simulink subsystem "Automatic_turn_light_feature_continuous_mdl"  (R2026a)
settings: Solver=VariableStepAuto
settings Model: Creator=irfan  LastModifiedBy=irfan

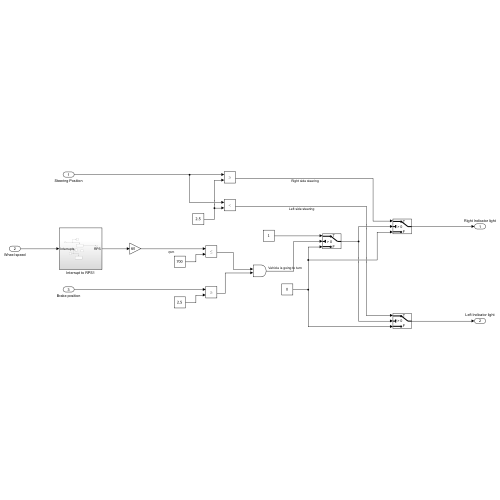
[thumbnail: Simulink's stored preview of the top-level diagram]
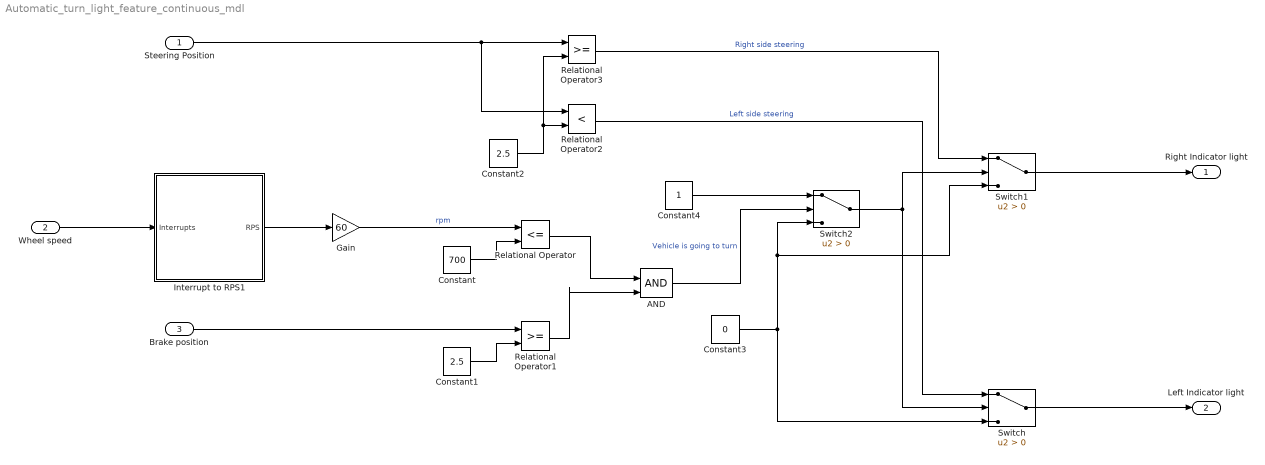
== system Automatic_turn_light_feature_continuous_mdl ==
  Steering Position : Inport
  Wheel speed : Inport  Port=2
  Brake position : Inport  Port=3
  AND : Logic  IconShape=distinctive  AllPortsSameDT=off  OutDataTypeStr=boolean
  Constant : Constant  Value=700
  Constant1 : Constant  Value=2.5
  Constant2 : Constant  Value=2.5
  Constant3 : Constant  Value=0
  Constant4 : Constant
  Gain : Gain  Gain=60
  Interrupt to RPS1 : Subsystem
  Relational Operator : RelationalOperator  Operator=<=  OutDataTypeStr=boolean  RndMeth=Simplest  InputSameDT=off
  Relational Operator1 : RelationalOperator  OutDataTypeStr=boolean  RndMeth=Simplest  InputSameDT=off
  Relational Operator2 : RelationalOperator  Operator=<  OutDataTypeStr=boolean  RndMeth=Simplest  InputSameDT=off
  Relational Operator3 : RelationalOperator  OutDataTypeStr=boolean  RndMeth=Simplest  InputSameDT=off
  Switch : Switch  Criteria=u2 > Threshold  SaturateOnIntegerOverflow=off  InputSameDT=off
  Switch1 : Switch  Criteria=u2 > Threshold  SaturateOnIntegerOverflow=off  InputSameDT=off
  Switch2 : Switch  Criteria=u2 > Threshold  SaturateOnIntegerOverflow=off  InputSameDT=off
  Right Indicator light : Outport
  Left Indicator light : Outport  Port=2
  wires:
  Relational Operator2/1 -> Switch/1  "Left side steering"
  Relational Operator1/1 -> AND/2
  Steering Position/1 -> Relational Operator3/1, Relational Operator2/1
  Constant2/1 -> Relational Operator2/2, Relational Operator3/2
  AND/1 -> Switch2/2  "Vehicle is going to turn"
  Constant3/1 -> Switch/3, Switch1/3, Switch2/3
  Constant4/1 -> Switch2/1
  Constant1/1 -> Relational Operator1/2
  Switch2/1 -> Switch/2, Switch1/2
  Constant/1 -> Relational Operator/2
  Gain/1 -> Relational Operator/1  "rpm"
  Relational Operator3/1 -> Switch1/1  "Right side steering"
  Relational Operator/1 -> AND/1
  Switch/1 -> Left Indicator light/1
  Switch1/1 -> Right Indicator light/1
  Brake position/1 -> Relational Operator1/1
  Wheel speed/1 -> Interrupt to RPS1/1(Interrupts)
  Interrupt to RPS1/1(RPS) -> Gain/1

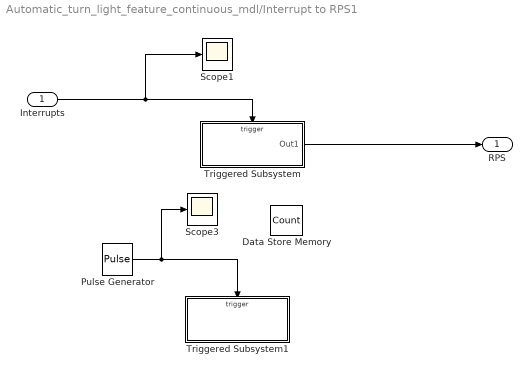
== system Automatic_turn_light_feature_continuous_mdl/Interrupt to RPS1 ==
  Interrupts : Inport
  Data Store Memory : DataStoreMemory  DataStoreName=Count  WriteAfterWriteMsg=warning  ShowAdditionalParam=off
  Pulse Generator : DiscretePulseGenerator  PulseType=Time based  Period=1.1  PulseWidth=10
  Scope1 : Scope
      settings: ActiveDisplayYMinimum=-0.13566588291136217  ActiveDisplayYMaximum=1.17702326681558
  Scope3 : Scope
      settings: ActiveDisplayYMinimum=-0.12499999999999997  ActiveDisplayYMaximum=1.125  DataLoggingVariableName=ScopeData2
  Triggered Subsystem : Subsystem  TreatAsAtomicUnit=on
  Triggered Subsystem1 : Subsystem  TreatAsAtomicUnit=on
  RPS : Outport
  wires:
  Interrupts/1 -> Triggered Subsystem/Trigger, Scope1/1
  Pulse Generator/1 -> Scope3/1, Triggered Subsystem1/Trigger
  Triggered Subsystem/1(Out1) -> RPS/1

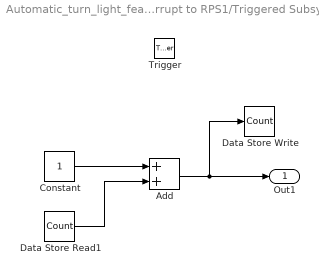
== system Automatic_turn_light_feature_continuous_mdl/Interrupt to RPS1/Triggered Subsystem ==
  Trigger : TriggerPort  VariantControl=(inherit)
  Add : Sum
  Constant : Constant  SampleTime=-1
  Data Store Read1 : DataStoreRead  DataStoreName=Count  IndexOptions=Index vector (dialog)  Indices=1  OutputSizes=1
  Data Store Write : DataStoreWrite  DataStoreName=Count  IndexOptions=Index vector (dialog)  Indices=1  OutputSizes=1
  Out1 : Outport
  wires:
  Add/1 -> Data Store Write/1, Out1/1
  Constant/1 -> Add/1
  Data Store Read1/1 -> Add/2

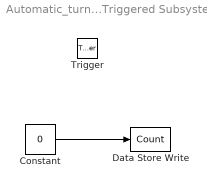
== system Automatic_turn_light_feature_continuous_mdl/Interrupt to RPS1/Triggered Subsystem1 ==
  Trigger : TriggerPort  VariantControl=(inherit)
  Constant : Constant  Value=0
  Data Store Write : DataStoreWrite  DataStoreName=Count  IndexOptions=Index vector (dialog)  Indices=1  OutputSizes=1
  wires:
  Constant/1 -> Data Store Write/1
